simulink model "F16ASYM_ControlledFAST"  (R2012b)
settings: Solver=ode4  SolverMode=SingleTasking  StartTime=0.0  StopTime=inf  FixedStep=T_sim  RelTol=1e-3
InitFcn:
  | mex nlplantASYM.c
values from neighbouring files (symbols this model uses):
  T_sim = 0.02    [RUN_ME.m]
undefined symbols (not defined in the file or in its folder): B, dLEF, Earth, fi_flag_Simulink, k_B, latitude, longitude, m, m_B, Model_used_flag, rad, s, sigbuilder_block, trim_control, trim_state, trim_throttle, WGS84
libraries: F16_Actuator_Library x14, simulink_extras x9, aerolibatmos2 x3, aerolibtransform2 x3, aerolibfltsims x3, aerolibconvert2 x2, dspmtrx3 x1, qcatlib x1, aerolibasang x1, aerolibanimutils x1, aerolibconvert x1, aerolibobsolete x1
(part 2 of 2)

== system F16ASYM_ControlledFAST/FlightGear visualization/Flat Earth to LLA ==
  note: Flat Earth to LLA
  Xe : Inport
  altitude0 : Inport  Port=2
  Angle Conversion : aerolibconvert2/Angle Conversion  IU=deg  OU=rad
  Demux2 : Demux  Outputs=2
  Demux6 : Demux  Outputs=[2 1]
  Display : Display
  Flat Earth to LLA : aerolibtransform2/Flat Earth to LLA  units=Metric (MKS)  ptype=Earth (WGS84)  F=1/298.257223563  R=6378137  LL0=[latitude longitude]  psi=0
  Gain : Gain  Gain=-1
  Mux : Mux  Inputs=2
  longitude l : Outport
  latitude mu : Outport  Port=2
  altitude h : Outport  Port=3
  wires:
  Flat Earth to LLA/1 -> Angle Conversion/1
  Demux2/1 -> latitude mu/1  "latitude"
  Demux2/2 -> longitude l/1
  Xe/1 -> Demux6/1
  altitude0/1 -> Flat Earth to LLA/2
  Flat Earth to LLA/2 -> Display/1, altitude h/1  "altitude"
  Angle Conversion/1 -> Demux2/1
  Mux/1 -> Flat Earth to LLA/1
  Demux6/1 -> Mux/1
  Demux6/2 -> Gain/1
  Gain/1 -> Mux/2

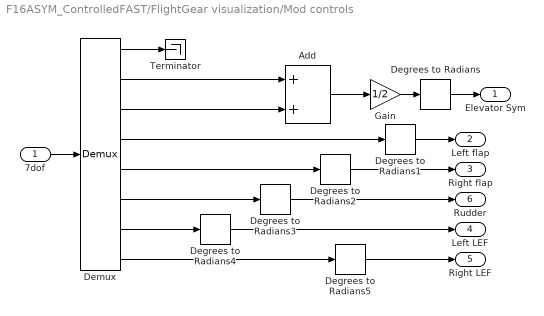
== system F16ASYM_ControlledFAST/FlightGear visualization/Mod controls ==
  "7dof " : Inport
  Add : Sum
  Degrees to Radians{,1..5} (6 alike) : simulink_extras/Transformations/Degrees to Radians
  Demux : Demux  Outputs=8
  Gain : Gain  Gain=1/2
  Terminator : Terminator
  Elevator Sym : Outport
  Left flap : Outport  Port=2
  Right flap : Outport  Port=3
  Left LEF : Outport  Port=4
  Right LEF : Outport  Port=5
  Rudder : Outport  Port=6
  wires:
  "7dof "/1 -> Demux/1
  Demux/2 -> Add/1
  Demux/3 -> Add/2
  Add/1 -> Gain/1
  Gain/1 -> Degrees to Radians/1
  Demux/4 -> Degrees to Radians1/1
  Demux/5 -> Degrees to Radians2/1
  Demux/6 -> Degrees to Radians3/1
  Demux/7 -> Degrees to Radians4/1
  Demux/8 -> Degrees to Radians5/1
  Demux/1 -> Terminator/1
  Degrees to Radians/1 -> Elevator Sym/1
  Degrees to Radians1/1 -> Left flap/1
  Degrees to Radians2/1 -> Right flap/1
  Degrees to Radians3/1 -> Rudder/1
  Degrees to Radians4/1 -> Left LEF/1
  Degrees to Radians5/1 -> Right LEF/1

== system F16ASYM_ControlledFAST/FlightGear visualization/phidot thetadot psidot ==
  pqr : Inport
  phi theta psi : Inport  Port=2
  Concatenate1 : Concatenate  NumInputs=3
  Concatenate2 : Concatenate  NumInputs=3
  SinCos : aerolibobsolete/SinCos
  keep angles in range [-pi pi] : Trigonometry  Operator=atan2
  phidot : Fcn  Expr=u[1]+(u[2]*u[4]+u[3]*u[7])*(u[5]/u[8])
  psidot : Fcn  Expr=(u[2]*u[4]+u[3]*u[7])/u[8]
  thetadot : Fcn  Expr=u[2]*u[7]-u[3]*u[4]
  ptp_earth : Outport
  ptp_dot : Outport  Port=2
  wires:
  SinCos/2 -> Concatenate1/3, keep angles in range [-pi pi]/2
  SinCos/1 -> Concatenate1/2, keep angles in range [-pi pi]/1
  Concatenate2/1 -> ptp_dot/1
  phidot/1 -> Concatenate2/1
  thetadot/1 -> Concatenate2/2
  psidot/1 -> Concatenate2/3
  phi theta psi/1 -> SinCos/1
  pqr/1 -> Concatenate1/1
  Concatenate1/1 -> thetadot/1, phidot/1, psidot/1
  keep angles in range [-pi pi]/1 -> ptp_earth/1

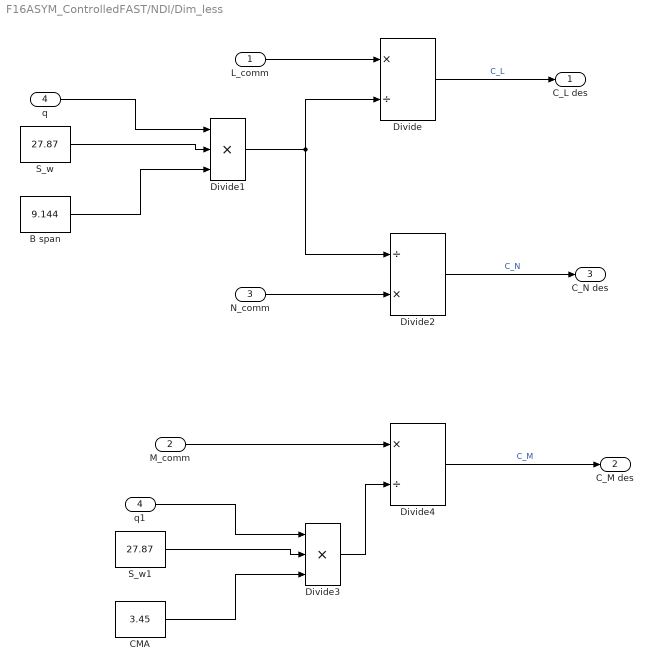
== system F16ASYM_ControlledFAST/NDI/Dim_less ==
  L_comm : Inport
  M_comm : Inport  Port=2
  N_comm : Inport  Port=3
  q : Inport  Port=4
  B span : Constant  Value=9.144
  CMA : Constant  Value=3.45
  Divide : Product  Inputs=*/
  Divide1 : Product  Inputs=***
  Divide2 : Product  Inputs=/*
  Divide3 : Product  Inputs=***
  Divide4 : Product  Inputs=*/
  S_w : Constant  Value=27.87
  S_w1 : Constant  Value=27.87
  q1 : InportShadow  Port=4
  C_L des : Outport
  C_M des : Outport  Port=2
  C_N des : Outport  Port=3
  wires:
  q/1 -> Divide1/1
  S_w/1 -> Divide1/2
  B span/1 -> Divide1/3
  L_comm/1 -> Divide/1
  Divide1/1 -> Divide2/1, Divide/2
  Divide/1 -> C_L des/1  "C_L"
  N_comm/1 -> Divide2/2
  Divide2/1 -> C_N des/1  "C_N"
  q1/1 -> Divide3/1
  S_w1/1 -> Divide3/2
  CMA/1 -> Divide3/3
  M_comm/1 -> Divide4/1
  Divide3/1 -> Divide4/2
  Divide4/1 -> C_M des/1  "C_M"

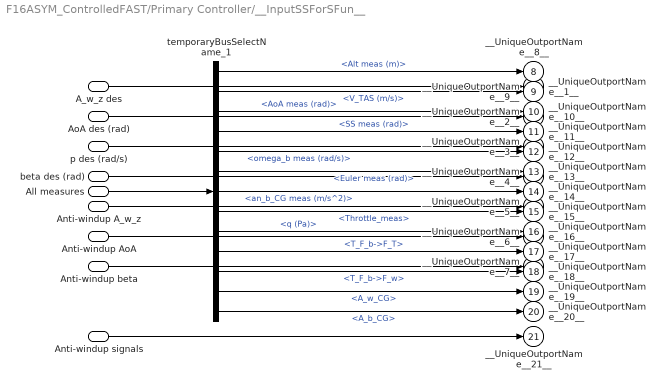
== system F16ASYM_ControlledFAST/Primary Controller/__InputSSForSFun__ ==
  A_w_z des : Inport
  AoA des (rad) : Inport  Port=2
  p des (rad/s) : Inport  Port=3
  beta des (rad) : Inport  Port=4
  Anti-windup A_w_z : Inport  Port=5
  Anti-windup AoA : Inport  Port=6
  Anti-windup beta : Inport  Port=7
  All measures : Inport  Port=8
  Anti-windup signals : Inport  Port=9
  temporaryBusSelectName_1 : BusSelector  OutputSignals=signal1.Alt meas (m),signal1.V_TAS (m/s),signal1.AoA meas (rad),signal1.SS meas (rad),signal1.omega_b meas (rad/s),signal1.Euler meas (rad),signal1.an_b_CG meas (m/s^2),signal1.Throttle_meas,signal2.q (Pa),signal2.T_F_b->F_T,signal2.T_F_b->F_w,signal2.A_w_CG,signal2.A_b_CG
  __UniqueOutportName__1__ : Outport
  __UniqueOutportName__2__ : Outport  Port=2
  __UniqueOutportName__3__ : Outport  Port=3
  __UniqueOutportName__4__ : Outport  Port=4
  __UniqueOutportName__5__ : Outport  Port=5
  __UniqueOutportName__6__ : Outport  Port=6
  __UniqueOutportName__7__ : Outport  Port=7
  __UniqueOutportName__8__ : Outport  Port=8
  __UniqueOutportName__9__ : Outport  Port=9
  __UniqueOutportName__10__ : Outport  Port=10
  __UniqueOutportName__11__ : Outport  Port=11
  __UniqueOutportName__12__ : Outport  Port=12
  __UniqueOutportName__13__ : Outport  Port=13
  __UniqueOutportName__14__ : Outport  Port=14
  __UniqueOutportName__15__ : Outport  Port=15
  __UniqueOutportName__16__ : Outport  Port=16
  __UniqueOutportName__17__ : Outport  Port=17
  __UniqueOutportName__18__ : Outport  Port=18
  __UniqueOutportName__19__ : Outport  Port=19
  __UniqueOutportName__20__ : Outport  Port=20
  __UniqueOutportName__21__ : Outport  Port=21
  wires:
  All measures/1 -> temporaryBusSelectName_1/1
  A_w_z des/1 -> __UniqueOutportName__1__/1
  AoA des (rad)/1 -> __UniqueOutportName__2__/1
  p des (rad/s)/1 -> __UniqueOutportName__3__/1
  beta des (rad)/1 -> __UniqueOutportName__4__/1
  Anti-windup A_w_z/1 -> __UniqueOutportName__5__/1
  Anti-windup AoA/1 -> __UniqueOutportName__6__/1
  Anti-windup beta/1 -> __UniqueOutportName__7__/1
  temporaryBusSelectName_1/1 -> __UniqueOutportName__8__/1  "<Alt meas (m)>"
  temporaryBusSelectName_1/2 -> __UniqueOutportName__9__/1  "<V_TAS (m/s)>"
  temporaryBusSelectName_1/3 -> __UniqueOutportName__10__/1  "<AoA meas (rad)>"
  temporaryBusSelectName_1/4 -> __UniqueOutportName__11__/1  "<SS meas (rad)>"
  temporaryBusSelectName_1/5 -> __UniqueOutportName__12__/1  "<omega_b meas (rad/s)>"
  temporaryBusSelectName_1/6 -> __UniqueOutportName__13__/1  "<Euler meas (rad)>"
  temporaryBusSelectName_1/7 -> __UniqueOutportName__14__/1  "<an_b_CG meas (m/s^2)>"
  temporaryBusSelectName_1/8 -> __UniqueOutportName__15__/1  "<Throttle_meas>"
  temporaryBusSelectName_1/9 -> __UniqueOutportName__16__/1  "<q (Pa)>"
  temporaryBusSelectName_1/10 -> __UniqueOutportName__17__/1  "<T_F_b->F_T>"
  temporaryBusSelectName_1/11 -> __UniqueOutportName__18__/1  "<T_F_b->F_w>"
  temporaryBusSelectName_1/12 -> __UniqueOutportName__19__/1  "<A_w_CG>"
  temporaryBusSelectName_1/13 -> __UniqueOutportName__20__/1  "<A_b_CG>"
  Anti-windup signals/1 -> __UniqueOutportName__21__/1

== system F16ASYM_ControlledFAST/Primary Controller/__OutputSSForSFun__ ==
  __UniqueInportName__1__ : Inport
  Angular acc des : Outport
  wires:
  __UniqueInportName__1__/1 -> Angular acc des/1

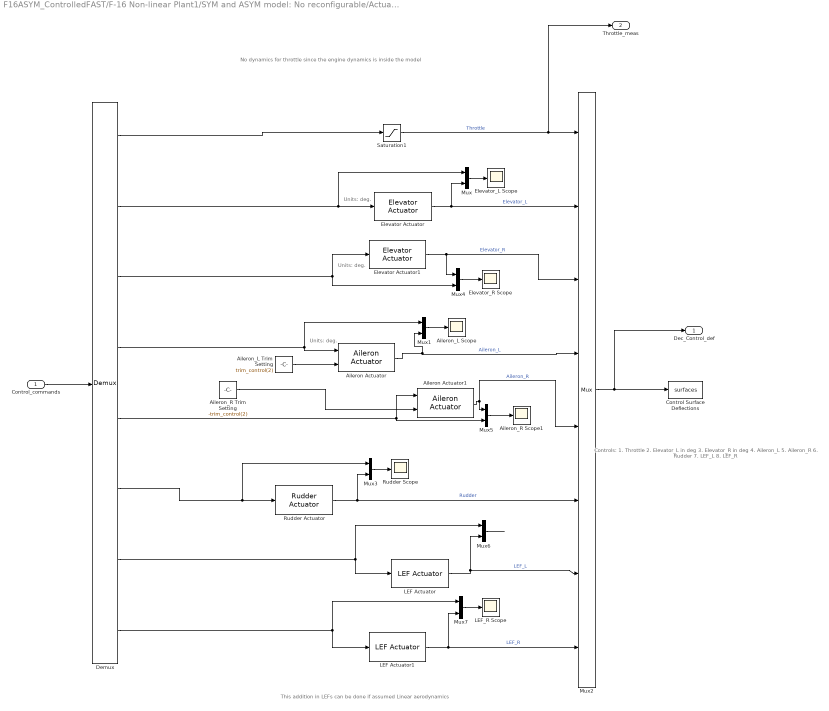
== system F16ASYM_ControlledFAST/F-16 Non-linear Plant1/SYM and ASYM model: No reconfigurable/Actuators Dynamcis ==
  note: Controls:
      | 1. Throttle
      | 2. Elevator_L in deg
      | 3. Elevator_R in deg
      | 4. Aileron_L
      | 5. Aileron_R
      | 6. Rudder
      | 7. LEF_L
      | 8. LEF_R
  note: Units: deg.
  note: Units: deg.
  note: Units: deg.
  note: This addition in LEFs can be done
      |  if assumed Linear aerodynamics
  note: No dynamics for throttle since the engine dynamics is inside the model
  Control_commands : Inport
  Aileron Actuator : F16_Actuator_Library/Aileron Actuator
  Aileron Actuator1 : F16_Actuator_Library/Aileron Actuator
  Aileron_L Scope : Scope
      settings: TimeRange=30  YMin=0  YMax=4.5  SaveName=ScopeData7
  Aileron_L Trim Setting : Constant  Value=trim_control(2)
  Aileron_R Scope1 : Scope
      settings: TimeRange=30  SaveName=ScopeData10
  Aileron_R Trim Setting : Constant  Value=-trim_control(2)
  Control Surface Deflections : ToWorkspace  VariableName=surfaces  SampleTime=-1
      settings: Decimation=100
  Demux : Demux  Outputs=8
  Elevator Actuator : F16_Actuator_Library/Elevator Actuator
  Elevator Actuator1 : F16_Actuator_Library/Elevator Actuator
  Elevator_L Scope : Scope
      settings: TimeRange=6  YMin=-2.1  YMax=-1.7  SaveName=ScopeData6
  Elevator_R Scope : Scope
      settings: TimeRange=4.5  YMin=-2.95  YMax=-2.4  SaveName=ScopeData9
  LEF Actuator : F16_Actuator_Library/LEF Actuator
  LEF Actuator1 : F16_Actuator_Library/LEF Actuator
  LEF_R Scope : Scope
      settings: YMin=5.75  YMax=5.92  SaveName=ScopeData12
  Mux{,1,3..7} (7 alike) : Mux  Inputs=2
  Mux2 : Mux  Inputs=8
  Rudder Actuator : F16_Actuator_Library/Rudder Actuator
  Rudder Scope : Scope
      settings: SaveName=ScopeData8
  Saturation1 : Saturate  UpperLimit=1  LowerLimit=0
  Dec_Control_def : Outport
  Throttle_meas : Outport  Port=2
  wires:
  Saturation1/1 -> Mux2/1, Throttle_meas/1  "Throttle"
  Aileron_R Trim Setting/1 -> Aileron Actuator1/2
  Aileron_L Trim Setting/1 -> Aileron Actuator/2
  Demux/1 -> Saturation1/1
  Mux7/1 -> LEF_R Scope/1
  LEF Actuator1/1 -> Mux7/2, Mux2/8  "LEF_R"
  Demux/8 -> Mux7/1, LEF Actuator1/1
  Mux6/1 -> ?
  LEF Actuator/1 -> Mux2/7, Mux6/2  "LEF_L"
  Demux/7 -> Mux6/1, LEF Actuator/1
  Mux5/1 -> Aileron_R Scope1/1
  Aileron Actuator1/1 -> Mux2/5, Mux5/1  "Aileron_R"
  Demux/5 -> Aileron Actuator1/1, Mux5/2
  Mux4/1 -> Elevator_R Scope/1
  Elevator Actuator1/1 -> Mux2/3, Mux4/1  "Elevator_R"
  Demux/3 -> Mux4/2, Elevator Actuator1/1
  Mux3/1 -> Rudder Scope/1
  Mux1/1 -> Aileron_L Scope/1
  Rudder Actuator/1 -> Mux2/6, Mux3/2  "Rudder"
  Aileron Actuator/1 -> Mux2/4, Mux1/2  "Aileron_L"
  Demux/6 -> Mux3/1, Rudder Actuator/1
  Demux/4 -> Aileron Actuator/1, Mux1/1
  Mux/1 -> Elevator_L Scope/1
  Elevator Actuator/1 -> Mux2/2, Mux/2  "Elevator_L"
  Mux2/1 -> Control Surface Deflections/1, Dec_Control_def/1
  Demux/2 -> Elevator Actuator/1, Mux/1
  Control_commands/1 -> Demux/1

== system F16ASYM_ControlledFAST/F-16 Non-linear Plant1/SYM and ASYM model: No reconfigurable/Leading Edge Flap:Symetric deflection ==
  note: Initialize LF_state with -alpha0 value in degrees!!!!
  note: Same as atmos() in nlplant...c
  note: see NASA Technical Paper 1538, p34
  state : Inport
  Bus Selector1 : BusSelector  OutputSignals=X_e,TAS,alpha;beta
  Creating    qbar / ps : Subsystem
  Demux : Demux  Outputs=3
  Demux1 : Demux  Outputs=2
  Gain : Gain  Gain=2  SaturateOnIntegerOverflow=on  OutDataTypeStr=Inherit: Same as input  ParamDataTypeStr=Inherit: Same as input
  Gain1 : Gain  Gain=7.25  SaturateOnIntegerOverflow=on  OutDataTypeStr=Inherit: Same as input  ParamDataTypeStr=Inherit: Same as input
  Gain2 : Gain  Gain=1.38  SaturateOnIntegerOverflow=on  OutDataTypeStr=Inherit: Same as input  ParamDataTypeStr=Inherit: Same as input
  LEF deflection : ToWorkspace  VariableName=d_LF  SampleTime=-1
      settings: Decimation=100
  LF_state : Integrator  InitialCondition=-trim_state(8)*180/pi
  Sum : Sum  Inputs=-|+|+  SaturateOnIntegerOverflow=on  InputSameDT=on  OutDataTypeStr=Inherit: Same as first input
  Sum1 : Sum  Inputs=|+-  SaturateOnIntegerOverflow=on  InputSameDT=on  OutDataTypeStr=Inherit: Same as first input
  Sum2 : Sum  Inputs=++|  SaturateOnIntegerOverflow=on  InputSameDT=on  OutDataTypeStr=Inherit: Same as first input
  coeff1 : Constant  Value=1.45
  r2d1 : Gain  Gain=180/pi  SaturateOnIntegerOverflow=on  OutDataTypeStr=Inherit: Same as input  ParamDataTypeStr=Inherit: Same as input
  r2d6 : Gain  Gain=9.05  SaturateOnIntegerOverflow=on  OutDataTypeStr=Inherit: Same as input  ParamDataTypeStr=Inherit: Same as input
  delta_lef (deg) : Outport
  wires:
  Bus Selector1/3 -> Demux1/1  "<alpha;beta>"
  Bus Selector1/1 -> Demux/1  "<X_e>"
  Demux/3 -> Creating    qbar / ps/1(alt)  "alt"
  r2d6/1 -> Sum/1
  Creating    qbar / ps/1(qbar / ps) -> r2d6/1
  Bus Selector1/2 -> Creating    qbar / ps/2(V)  "<TAS>"
  r2d1/1 -> Gain/1, Sum1/1  "alpha"
  LF_state/1 -> Sum2/2
  Sum2/1 -> Gain2/1, Sum1/2
  coeff1/1 -> Sum/3
  Demux1/1 -> r2d1/1
  Gain2/1 -> Sum/2
  Gain/1 -> Sum2/1
  Gain1/1 -> LF_state/1
  Sum1/1 -> Gain1/1
  state/1 -> Bus Selector1/1
  Sum/1 -> delta_lef (deg)/1, LEF deflection/1

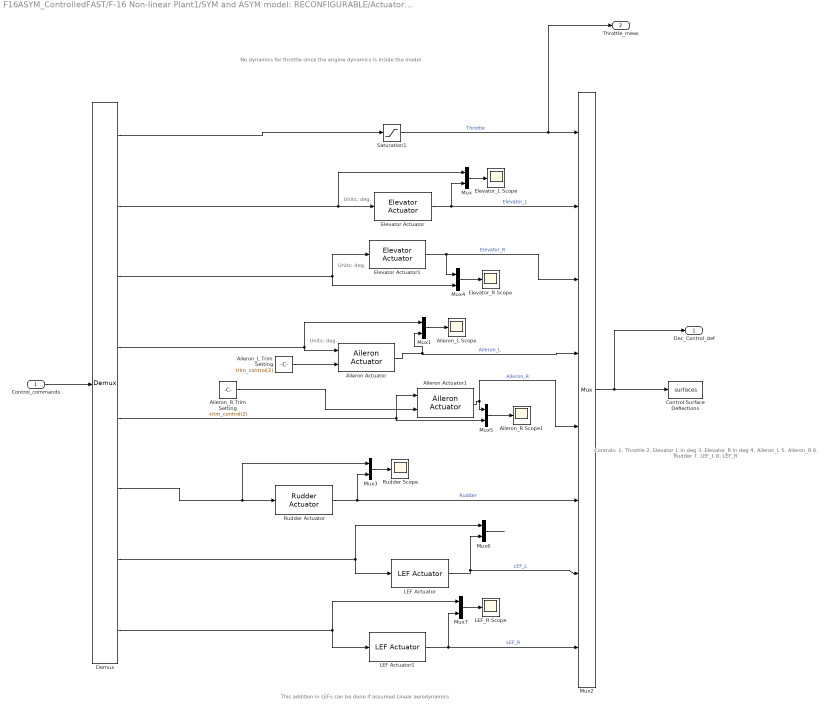
== system F16ASYM_ControlledFAST/F-16 Non-linear Plant1/SYM and ASYM model: RECONFIGURABLE/Actuators Dynamcis ==
  note: No dynamics for throttle since the engine dynamics is inside the model
  note: This addition in LEFs can be done
      |  if assumed Linear aerodynamics
  note: Units: deg.
  note: Units: deg.
  note: Units: deg.
  note: Controls:
      | 1. Throttle
      | 2. Elevator_L in deg
      | 3. Elevator_R in deg
      | 4. Aileron_L
      | 5. Aileron_R
      | 6. Rudder
      | 7. LEF_L
      | 8. LEF_R
  Control_commands : Inport
  Aileron Actuator : F16_Actuator_Library/Aileron Actuator
  Aileron Actuator1 : F16_Actuator_Library/Aileron Actuator
  Aileron_L Scope : Scope
      settings: TimeRange=30  YMin=0  YMax=4.5  SaveName=ScopeData7
  Aileron_L Trim Setting : Constant  Value=trim_control(2)
  Aileron_R Scope1 : Scope
      settings: TimeRange=30  SaveName=ScopeData10
  Aileron_R Trim Setting : Constant  Value=-trim_control(2)
  Control Surface Deflections : ToWorkspace  VariableName=surfaces  SampleTime=-1
      settings: Decimation=100
  Demux : Demux  Outputs=8
  Elevator Actuator : F16_Actuator_Library/Elevator Actuator
  Elevator Actuator1 : F16_Actuator_Library/Elevator Actuator
  Elevator_L Scope : Scope
      settings: TimeRange=5  YMin=-2.675  YMax=-2.125  SaveName=ScopeData6
  Elevator_R Scope : Scope
      settings: TimeRange=4.5  YMin=-2.95  YMax=-2.4  SaveName=ScopeData9
  LEF Actuator : F16_Actuator_Library/LEF Actuator
  LEF Actuator1 : F16_Actuator_Library/LEF Actuator
  LEF_R Scope : Scope
      settings: YMin=5.75  YMax=5.92  SaveName=ScopeData12
  Mux{,1,3..7} (7 alike) : Mux  Inputs=2
  Mux2 : Mux  Inputs=8
  Rudder Actuator : F16_Actuator_Library/Rudder Actuator
  Rudder Scope : Scope
      settings: SaveName=ScopeData8
  Saturation1 : Saturate  UpperLimit=1  LowerLimit=0
  Dec_Control_def : Outport
  Throttle_meas : Outport  Port=2
  wires:
  Control_commands/1 -> Demux/1
  Demux/2 -> Mux/1, Elevator Actuator/1
  Mux2/1 -> Dec_Control_def/1, Control Surface Deflections/1
  Elevator Actuator/1 -> Mux/2, Mux2/2  "Elevator_L"
  Mux/1 -> Elevator_L Scope/1
  Demux/4 -> Mux1/1, Aileron Actuator/1
  Demux/6 -> Rudder Actuator/1, Mux3/1
  Aileron Actuator/1 -> Mux1/2, Mux2/4  "Aileron_L"
  Rudder Actuator/1 -> Mux3/2, Mux2/6  "Rudder"
  Mux1/1 -> Aileron_L Scope/1
  Mux3/1 -> Rudder Scope/1
  Demux/3 -> Elevator Actuator1/1, Mux4/2
  Elevator Actuator1/1 -> Mux4/1, Mux2/3  "Elevator_R"
  Mux4/1 -> Elevator_R Scope/1
  Demux/5 -> Mux5/2, Aileron Actuator1/1
  Aileron Actuator1/1 -> Mux5/1, Mux2/5  "Aileron_R"
  Mux5/1 -> Aileron_R Scope1/1
  Demux/7 -> LEF Actuator/1, Mux6/1
  LEF Actuator/1 -> Mux6/2, Mux2/7  "LEF_L"
  Mux6/1 -> ?
  Demux/8 -> LEF Actuator1/1, Mux7/1
  LEF Actuator1/1 -> Mux2/8, Mux7/2  "LEF_R"
  Mux7/1 -> LEF_R Scope/1
  Demux/1 -> Saturation1/1
  Aileron_L Trim Setting/1 -> Aileron Actuator/2
  Aileron_R Trim Setting/1 -> Aileron Actuator1/2
  Saturation1/1 -> Throttle_meas/1, Mux2/1  "Throttle"

== system F16ASYM_ControlledFAST/F-16 Non-linear Plant1/SYM and ASYM model: RECONFIGURABLE/Leading Edge Flap:Symetric deflection ==
  note: see NASA Technical Paper 1538, p34
  note: Same as atmos() in nlplant...c
  note: Initialize LF_state with -alpha0 value in degrees!!!!
  state : Inport
  Bus Selector1 : BusSelector  OutputSignals=X_e,TAS,alpha;beta
  Creating    qbar / ps : Subsystem
  Demux : Demux  Outputs=3
  Demux1 : Demux  Outputs=2
  Gain : Gain  Gain=2  SaturateOnIntegerOverflow=on  OutDataTypeStr=Inherit: Same as input  ParamDataTypeStr=Inherit: Same as input
  Gain1 : Gain  Gain=7.25  SaturateOnIntegerOverflow=on  OutDataTypeStr=Inherit: Same as input  ParamDataTypeStr=Inherit: Same as input
  Gain2 : Gain  Gain=1.38  SaturateOnIntegerOverflow=on  OutDataTypeStr=Inherit: Same as input  ParamDataTypeStr=Inherit: Same as input
  LEF deflection : ToWorkspace  VariableName=d_LF  SampleTime=-1
      settings: Decimation=100
  LF_state : Integrator  InitialCondition=-trim_state(8)*180/pi
  Sum : Sum  Inputs=-|+|+  SaturateOnIntegerOverflow=on  InputSameDT=on  OutDataTypeStr=Inherit: Same as first input
  Sum1 : Sum  Inputs=|+-  SaturateOnIntegerOverflow=on  InputSameDT=on  OutDataTypeStr=Inherit: Same as first input
  Sum2 : Sum  Inputs=++|  SaturateOnIntegerOverflow=on  InputSameDT=on  OutDataTypeStr=Inherit: Same as first input
  coeff1 : Constant  Value=1.45
  r2d1 : Gain  Gain=180/pi  SaturateOnIntegerOverflow=on  OutDataTypeStr=Inherit: Same as input  ParamDataTypeStr=Inherit: Same as input
  r2d6 : Gain  Gain=9.05  SaturateOnIntegerOverflow=on  OutDataTypeStr=Inherit: Same as input  ParamDataTypeStr=Inherit: Same as input
  delta_lef (deg) : Outport
  wires:
  Sum/1 -> LEF deflection/1, delta_lef (deg)/1
  state/1 -> Bus Selector1/1
  Sum1/1 -> Gain1/1
  Gain1/1 -> LF_state/1
  Gain/1 -> Sum2/1
  Gain2/1 -> Sum/2
  Demux1/1 -> r2d1/1
  coeff1/1 -> Sum/3
  Sum2/1 -> Sum1/2, Gain2/1
  LF_state/1 -> Sum2/2
  r2d1/1 -> Sum1/1, Gain/1  "alpha"
  Bus Selector1/2 -> Creating    qbar / ps/2(V)  "<TAS>"
  Creating    qbar / ps/1(qbar / ps) -> r2d6/1
  r2d6/1 -> Sum/1
  Demux/3 -> Creating    qbar / ps/1(alt)  "alt"
  Bus Selector1/1 -> Demux/1  "<X_e>"
  Bus Selector1/3 -> Demux1/1  "<alpha;beta>"

== system F16ASYM_ControlledFAST/F-16 Non-linear Plant1/SYM and ASYM model: No reconfigurable/Leading Edge Flap:Symetric deflection/Creating    qbar // ps ==
  alt : Inport
  V : Inport  Port=2
  ISA Atmosphere Model : aerolibatmos2/ISA Atmosphere Model  custom=off  g=9.80665  gamma=1.4  R=287.0531  L=0.0065  h_trop=11000  h_strat=20000  rho0=1.225  P0=101325  T0=288.15
  Math Function1 : Math  Operator=square  SaturateOnIntegerOverflow=on
  Product : Product  Inputs=/*  SaturateOnIntegerOverflow=on  InputSameDT=on  OutDataTypeStr=Inherit: Same as first input
  Product5 : Product  Inputs=**  SaturateOnIntegerOverflow=on  InputSameDT=on  OutDataTypeStr=Inherit: Same as first input
  Terminator : Terminator
  Terminator1 : Terminator
  r2d4 : Gain  Gain=0.5  SaturateOnIntegerOverflow=on  OutDataTypeStr=Inherit: Same as input  ParamDataTypeStr=Inherit: Same as input
  qbar / ps : Outport
  wires:
  ISA Atmosphere Model/2 -> Terminator1/1
  ISA Atmosphere Model/1 -> Terminator/1
  ISA Atmosphere Model/3 -> Product/1
  ISA Atmosphere Model/4 -> Product5/1
  Product/1 -> qbar / ps/1
  V/1 -> Math Function1/1
  Product5/1 -> Product/2  "qbar"
  r2d4/1 -> Product5/2
  Math Function1/1 -> r2d4/1
  alt/1 -> ISA Atmosphere Model/1

== system F16ASYM_ControlledFAST/F-16 Non-linear Plant1/SYM and ASYM model: RECONFIGURABLE/Leading Edge Flap:Symetric deflection/Creating    qbar // ps ==
  alt : Inport
  V : Inport  Port=2
  ISA Atmosphere Model : aerolibatmos2/ISA Atmosphere Model  custom=off  g=9.80665  gamma=1.4  R=287.0531  L=0.0065  h_trop=11000  h_strat=20000  rho0=1.225  P0=101325  T0=288.15
  Math Function1 : Math  Operator=square  SaturateOnIntegerOverflow=on
  Product : Product  Inputs=/*  SaturateOnIntegerOverflow=on  InputSameDT=on  OutDataTypeStr=Inherit: Same as first input
  Product5 : Product  Inputs=**  SaturateOnIntegerOverflow=on  InputSameDT=on  OutDataTypeStr=Inherit: Same as first input
  Terminator : Terminator
  Terminator1 : Terminator
  r2d4 : Gain  Gain=0.5  SaturateOnIntegerOverflow=on  OutDataTypeStr=Inherit: Same as input  ParamDataTypeStr=Inherit: Same as input
  qbar / ps : Outport
  wires:
  alt/1 -> ISA Atmosphere Model/1
  Math Function1/1 -> r2d4/1
  r2d4/1 -> Product5/2
  Product5/1 -> Product/2  "qbar"
  V/1 -> Math Function1/1
  Product/1 -> qbar / ps/1
  ISA Atmosphere Model/4 -> Product5/1
  ISA Atmosphere Model/3 -> Product/1
  ISA Atmosphere Model/1 -> Terminator/1
  ISA Atmosphere Model/2 -> Terminator1/1

== matlab function F16ASYM_ControlledFAST/NDI/Pre-Inverter ==
  data: p_dot_comm input; L_comm output; q_dot_comm input; r_dot_comm input; M_comm output; N_comm output; omega_b input
function [L_comm,M_comm,N_comm] = Pre_inverter(p_dot_comm,q_dot_comm,r_dot_comm,omega_b)
Jy  = 75673.6;
Jxz = 1331.4; 
Jz  = 85552.1;  
Jx  = 12874.8;
h_E = 216.9;

Gamma = Jx * Jz - (Jxz  * Jxz);
C1 = ((Jy - Jz)  * Jz  - (Jxz * Jxz))/ Gamma;
C2 = ((Jx - Jy + Jz ) * Jxz ) / Gamma;
C3 = Jz / Gamma;
C4 = Jxz / Gamma;
C5 = (Jz - Jx) / Jy;
C6 = Jxz / Jy ;
C7 = 1 / Jy;
C8 = (Jx * (Jx - Jy ) + Jxz * Jxz) / Gamma;
C9 = Jx / Gamma;



L_comm = -( C4*r_dot_comm+(C2*C9-C4*C8)*omega_b(1)*omega_b(2)+(C2*C4+C1*C9)*omega_b(2)*omega_b(3)-C9*p_dot_comm )/(C3*C9-C4^2);

M_comm = (q_dot_comm-C5*omega_b(1)*omega_b(3)+C6*omega_b(1)^2-C6*omega_b(3)^2 +C7*h_E*omega_b(3))/C7;

N_comm = ( C3*r_dot_comm-C4*p_dot_comm+(C4*C1+C3*C2)*omega_b(2)*omega_b(3)+(C4*C2-C3*C8)*omega_b(1)*omega_b(2)+(C4^2-C3*C9)*h_E*omega_b(2) )/(C3*C9-C4^2);
